simulink model "driveKinematics"  (Simulink 7.7)
settings: Solver=ode45  StartTime=0.0  StopTime=10.0  RelTol=1e-3
values from neighbouring files (symbols this model uses):
  wheel_base = 0.5461    [horizon.m]    (also in robot.m; simulinkParams.m = 0.5; velocity_limits.m)
  wheel_radius = 0.159    [horizon.m]    (also in robot.m; simulinkParams.m = 0.1; velocity_limits.m)
settings Model: Creator=mjcarroll  LastModifiedBy=mjcarroll  TunableVars=initial_pose,wheel_base,wheel_radius  TunableVarsStorageClass=Auto,Auto,Auto  TunableVarsTypeQualifier=,,
settings OptimizationCC: InlineParams=on

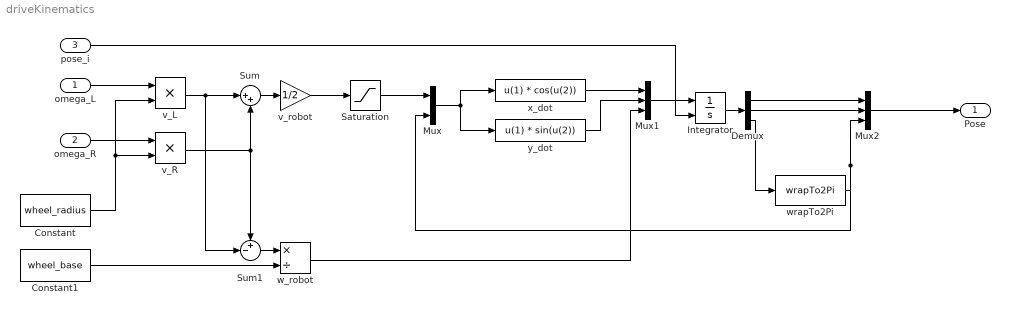
== system driveKinematics ==
  omega_L : Inport
  omega_R : Inport  Port=2
  pose_i : Inport  Port=3
  Constant : Constant  Value=wheel_radius  VectorParams1D=off
  Constant1 : Constant  Value=wheel_base  VectorParams1D=off
  Demux : Demux  Outputs=3
  Integrator : Integrator  InitialConditionSource=external  ContinuousStateAttributes='pose'
  Mux : Mux  Inputs=2
  Mux1 : Mux  Inputs=3
  Mux2 : Mux  Inputs=3
  Saturation : Saturate  UpperLimit=8  LowerLimit=-8
  Sum : Sum  Inputs=|++
  Sum1 : Sum  Inputs=+-|
  v_L : Product  RndMeth=Zero
  v_R : Product  RndMeth=Zero
  v_robot : Gain  Gain=1/2
  w_robot : Product  Inputs=*/
  wrapTo2Pi : MATLABFcn  MATLABFcn=wrapTo2Pi
  x_dot : Fcn  Expr=u(1) * cos(u(2))
  y_dot : Fcn  Expr=u(1) * sin(u(2))
  Pose : Outport
  wires:
  omega_L/1 -> v_L/1
  Constant/1 -> v_L/2, v_R/2
  omega_R/1 -> v_R/1
  v_L/1 -> Sum/1, Sum1/2
  v_R/1 -> Sum/2, Sum1/1
  Sum/1 -> v_robot/1
  Sum1/1 -> w_robot/1
  Constant1/1 -> w_robot/2
  Mux/1 -> x_dot/1, y_dot/1
  y_dot/1 -> Mux1/2
  x_dot/1 -> Mux1/1
  w_robot/1 -> Mux1/3
  Mux1/1 -> Integrator/1
  Integrator/1 -> Demux/1
  Demux/3 -> wrapTo2Pi/1
  Mux2/1 -> Pose/1
  wrapTo2Pi/1 -> Mux2/3, Mux/2
  Demux/1 -> Mux2/1
  Demux/2 -> Mux2/2
  pose_i/1 -> Integrator/2
  Saturation/1 -> Mux/1
  v_robot/1 -> Saturation/1
